simulink model "Active_Steering"  (R2020b)
settings: Solver=VariableStepAuto  StartTime=0.0  StopTime=10.0  RelTol=1e-3
undefined symbols (not defined in the file): sigbuilder_block
libraries: fl_lib x7, nesl_utility x4, sdl_lib x2, ee_lib x1, simulink x1
settings Model: Creator=sasad  LastModifiedBy=sasad

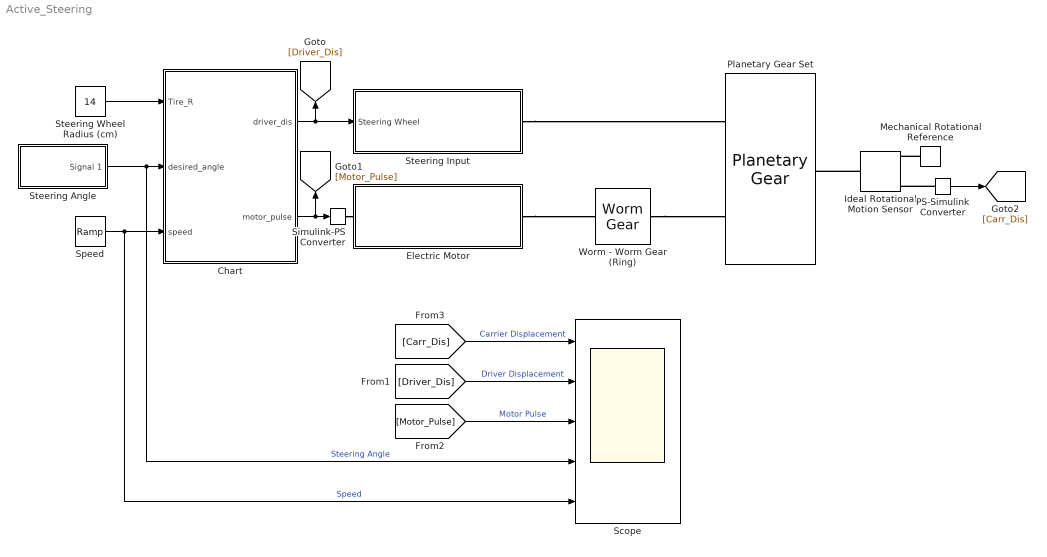
== system Active_Steering ==
  Chart : Stateflow chart  TreatAsAtomicUnit=on
  Electric Motor : Subsystem
  Ideal Rotational Motion Sensor : fl_lib/Mechanical/Mechanical Sensors/Ideal Rotational Motion Sensor  wrap_angle=simscape.enum.onoff.off  offset=0 rad
  Mechanical Rotational Reference : fl_lib/Mechanical/Rotational Elements/Mechanical Rotational Reference
  PS-Simulink Converter : nesl_utility/PS-Simulink Converter  PhysicalDomain=network_engine_domain  SubClassName=ps_output  LeftPortType=input  RightPortType=output  PseudoPeriodic=off  Frequencies=[]  Unit=inherit  AffineConversion=off
  Planetary Gear Set : sdl_lib/Gears/Planetary Gear  rs_ratio=2  friction_model=sdl.enum.gear_friction.none  mu_visc=[0, 0] N*m/(rad/s)  efficiency=[.96, .98]  temperature_TLU=[280, 300, 320] K  efficiency_sp_TLU=[.95, .9, .85]  efficiency_rp_TLU=[.95, .9, .85]  pwr_thr=[.001, .001] W  thermal_mass=50 J/K  T_init=300 K  model_inertia=simscape.enum.onoff.off  planet_inertia=0.001 kg*m^2
      settings: SourceProductBaseCode=LD
  Scope : Scope  NumInputPorts=5
  Simulink-PS Converter : nesl_utility/Simulink-PS Converter  PhysicalDomain=network_engine_domain  SubClassName=ps_input  LeftPortType=input  RightPortType=output  PseudoPeriodic=off  Frequencies=[]  NoiseDistribution=none  NoiseParameters=[]  Unit=1  AffineConversion=off  FilteringAndDerivatives=provide  SimscapeFilterOrder=1  InputFilterTimeConstant=0.001  UdotUserProvided=0
  Speed : simulink/Sources/Ramp  slope=10  start=0  InitialOutput=0
  Steering Angle : Subsystem  Tag=STV Subsys  LoadFcn=sigbuilder_block('load');  StartFcn=sigbuilder_block('start');  StopFcn=sigbuilder_block('stop');  ClipboardFcn=sigbuilder_block('clipboard');  mask(Sigbuilder block){tuvar=[0:10]}
      mask help: Simulink:masks:SigbuilderBlock_MD
      mask init:
      | if ~strcmp(get_param(bdroot(gcbh),'SimulationStatus'),'stopped') tuvar = sigbuilder_block('maskInit'); end
      settings: CopyFcn=sigbuilder_block('copy');  DeleteFcn=sigbuilder_block('delete');  ModelCloseFcn=sigbuilder_block('modelClose');  PreSaveFcn=sigbuilder_block('preSave');  PauseFcn=sigbuilder_block('pause');  ContinueFcn=sigbuilder_block('continue');  NameChangeFcn=sigbuilder_block('namechange');  OpenFcn=sigbuilder_block('open',[437.6 199.2 550.4 400 ]);  CloseFcn=sigbuilder_block('close');
      mask Display: plot(0, 0, 100, 100,[2, 2, 32, 32, 2], [68, 8, 8, 68, 68],[32, 2], [38, 38], [32, 19, 2],[53, 60, 44], [32, 17, 17, 2],[16, 16, 31, 31]);txt = getActiveGroup(gcbh);text(2, 100, txt,'verticalAlignment', 'top');
  Steering Input : Subsystem
  Steering Wheel Radius (cm) : Constant  Value=14
  Worm - Worm Gear (Ring) : sdl_lib/Gears/Worm Gear  ratio=30  thread_type=sdl.enum.handedness.right  friction_model=sdl.enum.gear_friction.none  mu_visc=[0, 0] N*m/(rad/s)  friction_parameterization=sdl.enum.efficiency_geometry.geometry  pr_ang=17.5 deg  lead_ang=20 deg  fr_coeff=0.08  eff_wg=0.74  eff_gw=0.65  temperature_TLU=[280, 300, 320] K  efficiency_wg_TLU=[.75, .65, .6]  efficiency_gw_TLU=[.5, .45, .4]  pwr_thr=0.001 W  thermal_mass=50 J/K  temperature_specify=off  temperature_priority=High  temperature=300 K  temperature_nominal_specify=off  temperature_nominal_unit=K  temperature_nominal_value=1
      settings: SourceProductBaseCode=LD  InternalSimscapePortConfiguration="{\"Bottom\":[],\"Left\":[{\"id\":\"W\",\"label\":\"W\",\"type\":\"foundation.mechanical.rotational.rotational\"}],\"Right\":[{\"id\":\"G\",\"label\":\"G\",\"type\":\"foundation.mechanical.rotational.rotational\"}],\"Top\":[]}"
  wires:
  Steering Wheel Radius (cm)/1 -> Chart/1(Tire_R)
  Steering Angle/1(Signal 1) -> Scope/4, Chart/2(desired_angle)  "Steering Angle"
  Speed/1 -> Scope/5, Chart/3(speed)  "Speed"
  Chart/1(driver_dis) -> Steering Input/1(Steering Wheel), [Driver_Dis]
  Chart/2(motor_pulse) -> [Motor_Pulse], Simulink-PS Converter/1
  PS-Simulink Converter/1 -> [Carr_Dis]
  [Carr_Dis] -> Scope/1  "Carrier Displacement"
  [Driver_Dis] -> Scope/2  "Driver Displacement"
  [Motor_Pulse] -> Scope/3  "Motor Pulse"
  connections:
  Worm - Worm Gear (Ring)/RConn1 -- Planetary Gear Set/RConn1
  Electric Motor/RConn1 -- Worm - Worm Gear (Ring)/LConn1
  Steering Input/RConn1 -- Planetary Gear Set/RConn2
  Ideal Rotational Motion Sensor/LConn1 -- Planetary Gear Set/LConn1
  Mechanical Rotational Reference/LConn1 -- Ideal Rotational Motion Sensor/RConn1
  Simulink-PS Converter/RConn1 -- Electric Motor/LConn1
  PS-Simulink Converter/LConn1 -- Ideal Rotational Motion Sensor/RConn3

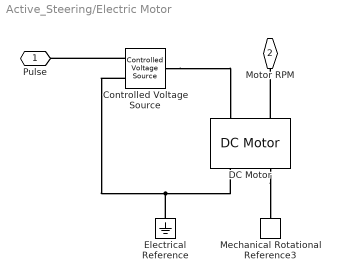
== system Active_Steering/Electric Motor ==
  Controlled Voltage Source : fl_lib/Electrical/Electrical Sources/Controlled Voltage Source
  DC Motor : ee_lib/Electromechanical/Brushed Motors/DC Motor  field_option=ee.enum.field_option.pm  Rf=100 Ohm  Lf=1 H  Laf=0.15 H  If0=0 A  parameterization=ee.enum.dcparam_option.circuit_param  Ra=3.9 Ohm  La=12e-6 H  emf_or_torque=ee.enum.emf_or_torque.kv  Kv=0.072e-3 V/rpm  Ki=6.876e-4 N*m/A  T_stall=0.24e-3 N*m  w_max=19100 rpm  w_rated=15000 rpm  P_rated=0.08 W  V_rated=1.5 V  J=0.01 g*cm^2  lam_param=ee.enum.lam_param.damping  lam=0 N*m/(rad/s)  i_noload=0 A  V_i_noload=1.5 V  speed0=0 rpm  enable_fault_armature=ee.enum.faults.faultEnable.no  rev_faulted=1 / 3  G_faulted_armature=1e-5 S  fault_trigger_armature=ee.enum.faults.faultTrigger.temporal  t_fault_armature=1 s  max_permissible_current_armature=inf A  t_fail_on_current_armature=1 s  enable_fault_field=ee.enum.faults.faultEnable.no  G_faulted_field=1e-5 S  fault_trigger_field=ee.enum.faults.faultTrigger.temporal  t_fault_field=1 s  max_permissible_current_field=inf A  t_fail_on_current_field=1 s  fault_action=ee.enum.faults.faultAction.none  alpha=3.93e-3 1/K  Tmeas=25 degC  thermal_mass=100 J/K  initial_temperature=25 degC
  Electrical Reference : fl_lib/Electrical/Electrical Elements/Electrical Reference
  Mechanical Rotational Reference3 : fl_lib/Mechanical/Rotational Elements/Mechanical Rotational Reference
  Pulse : PMIOPort  Side=Left
  Motor RPM : PMIOPort  Port=2  Side=Right
  connections:
  DC Motor/LConn2 -- Motor RPM/RConn1
  DC Motor/RConn2 -- Mechanical Rotational Reference3/LConn1
  Controlled Voltage Source/LConn1 -- DC Motor/LConn1
  Electrical Reference/LConn1 -- DC Motor/RConn1 -- Controlled Voltage Source/RConn2
  Controlled Voltage Source/RConn1 -- Pulse/RConn1

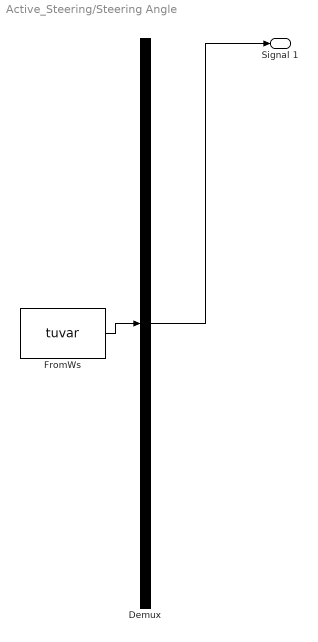
== system Active_Steering/Steering Angle ==
  Demux : Demux  Tag=STV Demux  Outputs=1
      settings: DisplayOption=none
  FromWs : FromWorkspace  Tag=STV FromWs  VariableName=tuvar
      SigBuilderData=|
      | common.afterFinalStr = 'Extrapolate'
      | common.sampleTime = 0
      | dataSet.timeRange = [0 10]
      | dataSet.name = 'Group 1'
      | sbobj.Groups.Name = 'Group 1'
      | sbobj.Groups.Signals.Name = 'Signal 1'
      | sbobj.Groups.Signals.XData = [0 4 7 7 10]
      | sbobj.Groups.Signals.YData = [0 0 80 0 0]
  Signal 1 : Outport  Tag=STV Outport
  wires:
  Demux/1 -> Signal 1/1
  FromWs/1 -> Demux/1

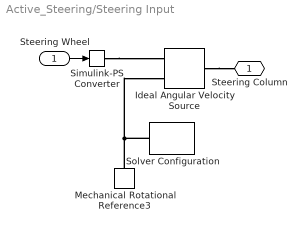
== system Active_Steering/Steering Input ==
  Steering Wheel : Inport
  Ideal Angular Velocity Source : fl_lib/Mechanical/Mechanical Sources/Ideal Angular Velocity Source
  Mechanical Rotational Reference3 : fl_lib/Mechanical/Rotational Elements/Mechanical Rotational Reference
  Simulink-PS Converter : nesl_utility/Simulink-PS Converter  PhysicalDomain=network_engine_domain  SubClassName=ps_input  LeftPortType=input  RightPortType=output  PseudoPeriodic=off  Frequencies=[]  NoiseDistribution=none  NoiseParameters=[]  Unit=1  AffineConversion=off  FilteringAndDerivatives=provide  SimscapeFilterOrder=1  InputFilterTimeConstant=0.001  UdotUserProvided=0
  Solver Configuration : nesl_utility/Solver Configuration  PhysicalDomain=network_engine_domain  SubClassName=solver  LeftPortType=input  RightPortType=generic  Tones=[]  Harmonics=[]  SimulateNoise=off  Profile=off  UseLocalSampling=off  EnableSwitchedLinearOptims=on  FrequencyDomain=off  UseCCode=off  RelTol=0.001  AbsTol=1e-06  MinStep=1e-09  ToWorkspace=off  RevertToSquareIcSolve=off  NumHomotopyIterations=100  PhasorMode=off  PhasorModeNumHarmonics=1  DoDC=off  ResidualTolerance=1e-09  UseLocalSolver=off  LocalSolverChoice=NE_BACKWARD_EULER_ADVANCER  LocalSolverSampleTime=0.001  DoFixedCost=off  MaxNonlinIter=3  MaxModeIter=2  ComputeImpulses=off  ImpulseIterations=2  LinearAlgebra=auto  EquationFormulation=NE_TIME_EF  DelaysMemoryBudget=1024  AutomaticFiltering=on  FilteringTimeConstant=0.001  PartitionStorageMethod=AS_NEEDED  PartitionMemoryBudget=1024  PartitionMethod=ROBUST
  Steering Column : PMIOPort  Side=Right
  wires:
  Steering Wheel/1 -> Simulink-PS Converter/1
  connections:
  Ideal Angular Velocity Source/LConn1 -- Steering Column/RConn1
  Simulink-PS Converter/RConn1 -- Ideal Angular Velocity Source/RConn1
  Mechanical Rotational Reference3/LConn1 -- Solver Configuration/RConn1 -- Ideal Angular Velocity Source/RConn2

== stateflow chart Active_Steering/Chart ==
  state Assist
    du:
    help_ratio = ((60-speed)/60) * 0.3;
    driver_angle = floor(desired_angle*(1-help_ratio));
    motor_angle = ceil(desired_angle*help_ratio);
    driver_dis = Tire_R*driver_angle*pi/180;
    motor_dis = Tire_R*motor_angle*pi/180;
    motor_pulse = 1;
  state Start
  state Resist
    du:
    res_ratio = ((speed-60)/160) * 0.3;
    driver_angle = floor(desired_angle*(1-res_ratio));
    motor_angle = ceil(desired_angle*res_ratio);
    driver_dis = Tire_R*driver_angle*pi/180;
    motor_dis = Tire_R*motor_angle*pi/180;
    motor_pulse = -1;
  (default) -> Start
  Start -> Assist [order 1] : [speed <= 60]
  Assist -> Resist : [speed > 60]
  Resist -> Assist : [speed <= 60]
  Start -> Resist [order 2] : [speed > 60]
  data: Tire_R input; desired_angle input; speed input; driver_dis output; driver_angle local; help_ratio local; motor_angle local; res_ratio local; motor_pulse output; motor_dis local
